simulink model "d_IMU"  (R2015a)
settings: Solver=ode45  StartTime=0.0  StopTime=10.0  RelTol=1e-3
settings Model: CovSFcnEnable=off  Creator=Mattia  LastModifiedBy=pela
settings DebuggingCC: SolverPrmCheckMsg=warning

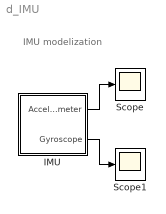
== system d_IMU ==
  note: IMU modelization
  IMU : Subsystem
  Scope : Scope
      settings: ShowLegends=on
  Scope1 : Scope
      settings: ShowLegends=on
  wires:
  IMU/2(Gyroscope) -> Scope1/1
  IMU/1(Accelerometer) -> Scope/1

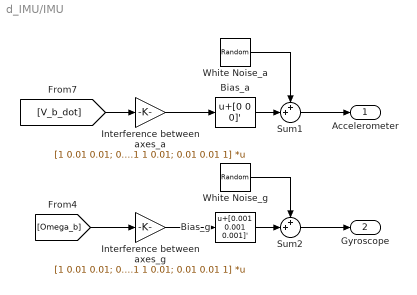
== system d_IMU/IMU ==
  Bias_a : Bias  Bias=[0 0 0]'
  Bias_g : Bias  Bias=[0.001 0.001 0.001]'
  Interference between axes_a : Gain  Gain=[1 0.01 0.01; 0.01 1 0.01; 0.01 0.01 1]  Multiplication=Matrix(K*u)
  "Interference between axes_g " : Gain  Gain=[1 0.01 0.01; 0.01 1 0.01; 0.01 0.01 1]  Multiplication=Matrix(K*u)
  Sum1 : Sum  Inputs=++|
  Sum2 : Sum  Inputs=++|
  White Noise_a : RandomNumber  DisableCoverage=on  Variance=0.0001  SampleTime=0.01
  White Noise_g : RandomNumber  DisableCoverage=on  Variance=0.0001  SampleTime=0.01
  Accelerometer : Outport
  Gyroscope : Outport  Port=2
  wires:
  White Noise_a/1 -> Sum1/1
  [Omega_b] -> "Interference between axes_g "/1
  Sum1/1 -> Accelerometer/1
  "Interference between axes_g "/1 -> Bias_g/1
  Interference between axes_a/1 -> Bias_a/1
  Bias_g/1 -> Sum2/2
  White Noise_g/1 -> Sum2/1
  Bias_a/1 -> Sum1/2
  Sum2/1 -> Gyroscope/1
  [V_b_dot] -> Interference between axes_a/1
